simulink model "Modell_V3"  (R2015b)
settings: Solver=ode45  StartTime=0.0  StopTime=0.5  RelTol=1e-3
values from neighbouring files (symbols this model uses):
  AP = modelPars(ii).AP    [Hilfsskript_sFunction.m]
  K = berechneLQR(A,B,Q,R)    [Hilfsskript_sFunction.m]
  M_AP = double(M_AP)    [linearisierung.m]
  stPendel = ladePendel    [Hilfsskript_sFunction.m]
  x0 = modelPars(ii).x0    [Hilfsskript_sFunction.m]
settings Model: Creator=asacakli  LastModifiedBy=ajentsch

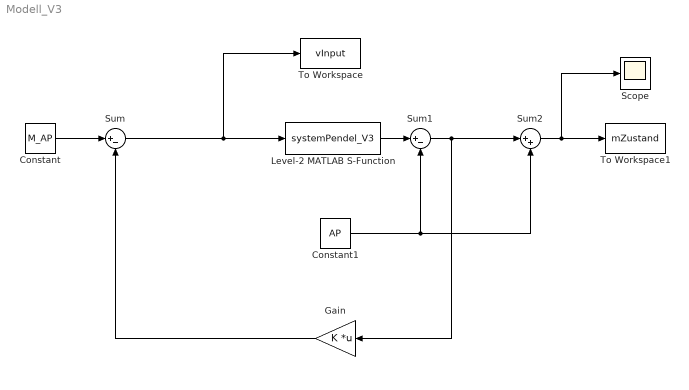
== system Modell_V3 ==
  Constant : Constant  Value=M_AP
  Constant1 : Constant  Value=AP
  Gain : Gain  Gain=K  Multiplication=Matrix(K*u)
  Level-2 MATLAB S-Function : M-S-Function  FunctionName=systemPendel_V3  Parameters=stPendel,x0
  Scope : Scope
  Sum : Sum  Inputs=|+-
  Sum1 : Sum  Inputs=|+-
  Sum2 : Sum  Inputs=|++
  To Workspace : ToWorkspace  VariableName=vInput  SaveFormat=Timeseries  SampleTime=-1
  To Workspace1 : ToWorkspace  VariableName=mZustand  SaveFormat=Timeseries  SampleTime=-1
  wires:
  Constant/1 -> Sum/1
  Gain/1 -> Sum/2
  Sum/1 -> To Workspace/1, Level-2 MATLAB S-Function/1
  Sum1/1 -> Sum2/1, Gain/1
  Constant1/1 -> Sum2/2, Sum1/2
  Level-2 MATLAB S-Function/1 -> Sum1/1
  Sum2/1 -> Scope/1, To Workspace1/1
